simulink model "pendsim"  (R2016a)
settings: Solver=FixedStepAuto  StartTime=t(N+1)  StopTime=t(end-N)  FixedStep=T  MaxStep=0.01  RelTol=1e-3
values from neighbouring files (symbols this model uses):
  c = 0.0044    [Q2_3.m]    (also in pend_lsqf.m = Res(2); pend_optimum.m = res(2))
  dtheta = y(2)    [pend_cost.m]    (also in pend_optimum.m = zeros(HIGHDATA - LOWDATA - 2*N + 1, size(data,1)); pend_plot.m)
  g = 9.81    [pend_optimum.m]
  I = 0.0092    [Q2_3.m]    (also in pend_lsqf.m = Res(1); pend_optimum.m = res(1))
  l = 95e-3    (= 0.095)    [pend_optimum.m]
  M = 552e-3    (= 0.552)    [pend_optimum.m]
  N = 23    [Q2_3.m]    (also in minimiseMotorCost.m = 17; motor_freeinertia.m = 17; motor_freerun.m; motor_plot_load.m = 17)
  theta = y(1)    [pend_cost.m]    (also in pend_optimum.m = zeros(HIGHDATA - LOWDATA - 2*N + 1, size(data,1)); pend_plot.m)
settings Model: Creator=masom  LastModifiedBy=masom
settings DataIOCC: ExternalInput=[I, c, M, g, l]  SaveOutput=off  SaveTime=off

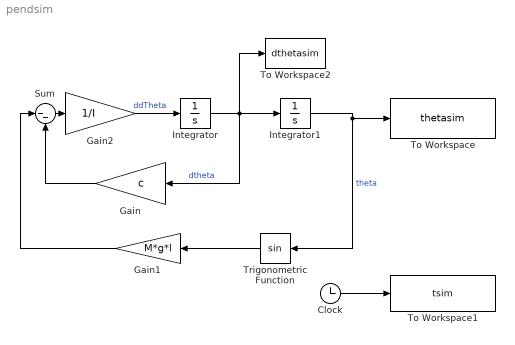
== system pendsim ==
  Clock : Clock
  Gain : Gain  Gain=c
  Gain1 : Gain  Gain=M*g*l
  Gain2 : Gain  Gain=1/I
  Integrator : Integrator  InitialCondition=dtheta(N+1)
  Integrator1 : Integrator  InitialCondition=theta(N+1)
  Sum : Sum  Inputs=|--
  To Workspace : ToWorkspace  VariableName=thetasim  SampleTime=-1
  To Workspace1 : ToWorkspace  VariableName=tsim  SampleTime=-1
  To Workspace2 : ToWorkspace  VariableName=dthetasim  SampleTime=-1
  Trigonometric Function : Trigonometry
  wires:
  Integrator/1 -> To Workspace2/1, Gain/1, Integrator1/1  "dtheta"
  Integrator1/1 -> Trigonometric Function/1, To Workspace/1  "theta"
  Sum/1 -> Gain2/1
  Gain/1 -> Sum/2
  Gain1/1 -> Sum/1
  Trigonometric Function/1 -> Gain1/1
  Clock/1 -> To Workspace1/1
  Gain2/1 -> Integrator/1  "ddTheta"
